simulink model "VelocidadeComoEntradaNoBlocoMotor"  (R2024b)
settings: Solver=VariableStepAuto  StartTime=0.0  StopTime=10  RelTol=1e-3
undefined symbols (not defined in the file): AirTemperature, C1, C2, C3, EV, fractalcoef, MTR, VelRef
libraries: vehdynlibtire x4, autolibmappedmotor x2, vrlib x1, slpidlib x1, mspsensorlib x1, vehdynlibviscommon x1, vehdynlibscenariocommon x1, vehdynlibsuspension x1, vehdynlibsteering x1, vehdynlibdriver x1, autolibshared x1
(part 1 of 3)
settings Model: SimulationMode=accelerator  Creator=João Gabriel  LastModifiedBy=João Gabriel
settings SolverCC: ZeroCrossAlgorithm=Adaptive
settings DebuggingCC: IgnoredZcDiagnostic=none

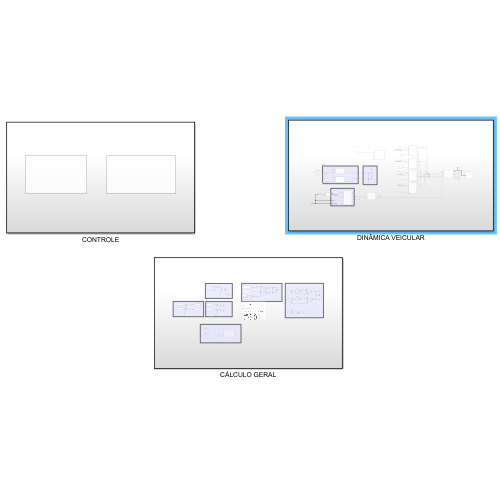
[thumbnail: Simulink's stored preview of the top-level diagram]
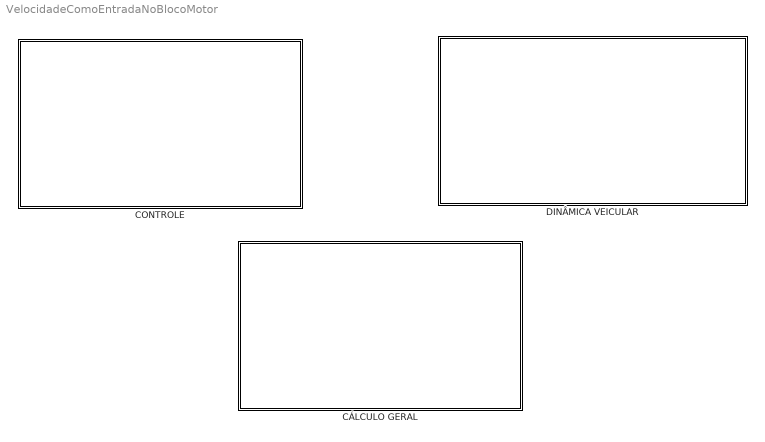
== system VelocidadeComoEntradaNoBlocoMotor ==
  CONTROLE : Subsystem
  CÁLCULO GERAL : Subsystem
  DINÂMICA VEICULAR : Subsystem

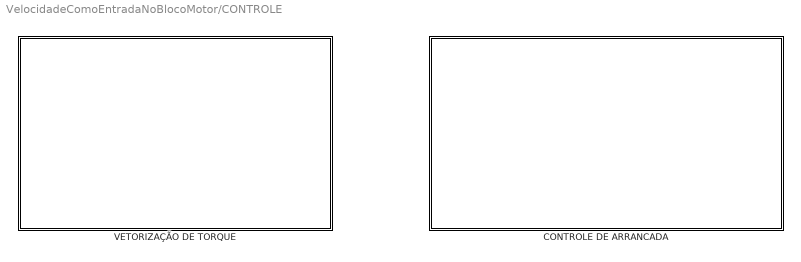
== system VelocidadeComoEntradaNoBlocoMotor/CONTROLE ==
  "CONTROLE DE ARRANCADA " : Subsystem
  "VETORIZAÇÃO DE TORQUE " : Subsystem

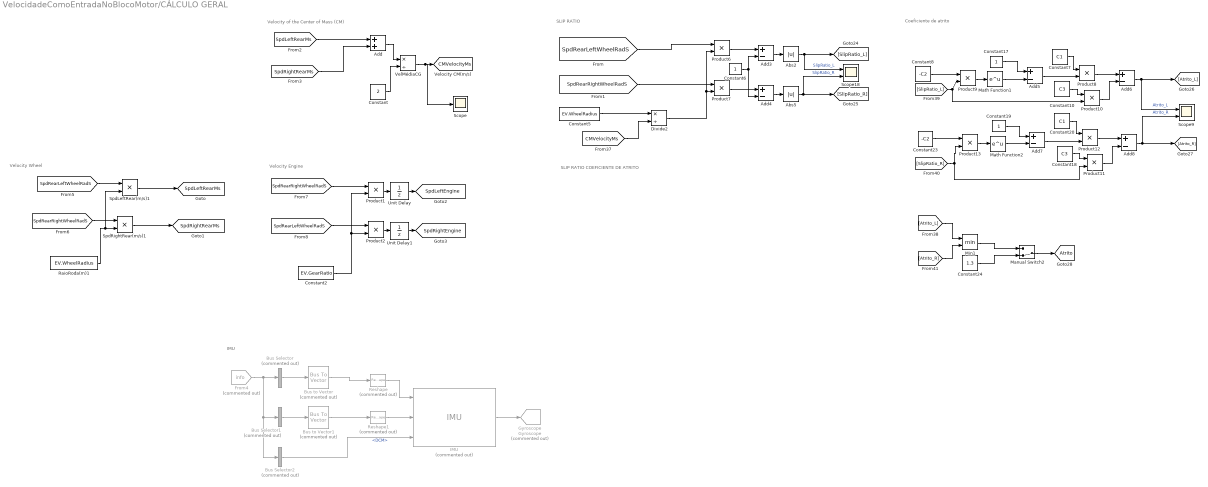
== system VelocidadeComoEntradaNoBlocoMotor/CÁLCULO GERAL ==
  note: Velocity Wheel
  note: Velocity Engine
  note: IMU
  note: Velocity of the Center of Mass (CM)
  note: SLIP RATIO
  note: Coeficiente de atrito
  note: SLIP RATIO
      |
      | COEFICIENTE DE ATRITO
  Abs2 : Abs  SaturateOnIntegerOverflow=off
  Abs5 : Abs  SaturateOnIntegerOverflow=off
  Add : Sum
  Add{3..8} (6 alike) : Sum  Inputs=+-
  Bus Selector : BusSelector  Commented=on  OutputSignals=BdyFrm.Cg.Acc.zddot,BdyFrm.Cg.Acc.yddot,BdyFrm.Cg.Acc.xddot  OutputAsBus=on
  Bus Selector1 : BusSelector  Commented=on  OutputSignals=BdyFrm.Cg.AngVel.p,BdyFrm.Cg.AngVel.q,BdyFrm.Cg.AngVel.r  OutputAsBus=on
  Bus Selector2 : BusSelector  Commented=on  OutputSignals=BdyFrm.Cg.DCM
  Bus to Vector : BusToVector  Commented=on
  Bus to Vector1 : BusToVector  Commented=on
  Constant : Constant  Value=2
  Constant10 : Constant  Value=C3
  Constant17 : Constant
  Constant18 : Constant  Value=C3
  Constant19 : Constant
  Constant2 : Constant  Value=EV.GearRatio
  Constant20 : Constant  Value=C1
  Constant23 : Constant  Value=-C2
  Constant24 : Constant  Value=1.3  VectorParams1D=off
  Constant5 : Constant  Value=EV.WheelRadius  VectorParams1D=off
  Constant6 : Constant
  Constant7 : Constant  Value=C1
  Constant8 : Constant  Value=-C2
  Divide2 : Product  Inputs=*/
  From4 : From  Commented=on  GotoTag=info  TagVisibility=global
  "Gyroscope " : Goto  Commented=on  GotoTag=Gyroscope  TagVisibility=global
  IMU : mspsensorlib/IMU  Commented=on  DispRefFrame=NED  TemperaturePort=off  Temperature=25  MagneticFieldPort=off  MagneticFieldNED=[ 27.5550, -2.4169, -16.0849 ]  MagneticFieldENU=[ -2.4169, 27.5550, 16.0849 ]  SeedDouble=67  SimulateUsing=Interpreted execution  AccelParamsMeasurementRange=Inf  AccelParamsResolution=0  AccelParamsConstantBias=[ 0, 0, 0 ]  AccelParamsAxesMisalignment=[ 100, 0, 0; 0, 100, 0; 0, 0, 100 ]  AccelParamsNoiseDensity=[ 0, 0, 0 ]  AccelParamsBiasInstability=[ 0, 0, 0 ]  AccelParamsBiasInstabilityNumerator=fractalcoef().Numerator  AccelParamsBiasInstabilityDenominator=fractalcoef().Denominator  AccelParamsRandomWalk=[ 0, 0, 0 ]  AccelParamsNoiseType=double-sided  AccelParamsTemperatureBias=[ 0, 0, 0 ]  AccelParamsTemperatureScaleFactor=[ 0, 0, 0 ]  GyroParamsMeasurementRange=Inf  GyroParamsResolution=0  GyroParamsConstantBias=[ 0, 0, 0 ]  GyroParamsAxesMisalignment=[ 100, 0, 0; 0, 100, 0; 0, 0, 100 ]  GyroParamsAccelerationBias=[ 0, 0, 0 ]  GyroParamsNoiseDensity=[ 0, 0, 0 ]  GyroParamsBiasInstability=[ 0, 0, 0 ]  GyroParamsBiasInstabilityNumerator=fractalcoef().Numerator  GyroParamsBiasInstabilityDenominator=fractalcoef().Denominator  GyroParamsRandomWalk=[ 0, 0, 0 ]  GyroParamsNoiseType=double-sided  GyroParamsTemperatureBias=[ 0, 0, 0 ]  GyroParamsTemperatureScaleFactor=[ 0, 0, 0 ]  MagParamsMeasurementRange=Inf  MagParamsResolution=0  MagParamsConstantBias=[ 0, 0, 0 ]  MagParamsAxesMisalignment=[ 100, 0, 0; 0, 100, 0; 0, 0, 100 ]  MagParamsNoiseDensity=[ 0, 0, 0 ]  MagParamsBiasInstability=[ 0, 0, 0 ]  MagParamsBiasInstabilityNumerator=fractalcoef().Numerator  MagParamsBiasInstabilityDenominator=fractalcoef().Denominator  MagParamsRandomWalk=[ 0, 0, 0 ]  MagParamsNoiseType=double-sided  MagParamsTemperatureBias=[ 0, 0, 0 ]  MagParamsTemperatureScaleFactor=[ 0, 0, 0 ]
  Manual Switch2 : ManualSwitch  CurrentSetting=0
  Math Function1 : Math
  Math Function2 : Math
  Min1 : MinMax  Inputs=2
  Product{1..2,6..13} (10 alike) : Product
  RaioRoda(m)1 : Constant  Value=EV.WheelRadius  VectorParams1D=off
  Reshape : Reshape  Commented=on  OutputDimensionality=Customize  OutputDimensions=[1,3]
  Reshape1 : Reshape  Commented=on  OutputDimensionality=Customize  OutputDimensions=[1,3]
  Scope : Scope
  Scope18 : Scope  NumInputPorts=2
  Scope9 : Scope  NumInputPorts=2
  SpdLeftRear(m/s)1 : Product
  SpdRightRear(m/s)1 : Product
  Unit Delay : UnitDelay  SampleTime=-1  HasFrameUpgradeWarning=on
  Unit Delay1 : UnitDelay  SampleTime=-1  HasFrameUpgradeWarning=on
  VelMédiaCG : Product  Inputs=*/
  tag scope: Atrito=global, CMVelocityMs=global, SpdLeftEngine=global, SpdLeftRearMs=global, SpdRightEngine=global, SpdRightRearMs=global
  wires:
  Constant6/1 -> Add3/2, Add4/2
  Add6/1 -> Scope9/1, [Atrito_L]  "Atrito_L"
  Abs2/1 -> Scope18/1, [SlipRatio_L]  "SlipRatio_L"
  Constant7/1 -> Product8/1
  Constant19/1 -> Add7/1
  Constant24/1 -> Manual Switch2/2
  Constant23/1 -> Product13/1
  Add4/1 -> Abs5/1
  Add3/1 -> Abs2/1
  Product11/1 -> Add8/2
  Abs5/1 -> Scope18/2, [SlipRatio_R]  "SlipRatio_R"
  Product12/1 -> Add8/1
  Product10/1 -> Add6/2
  Product8/1 -> Add6/1
  Math Function2/1 -> Add7/2
  Add7/1 -> Product12/2
  [Atrito_L] -> Min1/1
  Constant10/1 -> Product10/1
  Math Function1/1 -> Add5/2
  Constant18/1 -> Product11/1
  [SlipRatio_L] -> Product10/2, Product9/2
  Add8/1 -> Scope9/2, [Atrito_R]  "Atrito_R"
  Product9/1 -> Math Function1/1
  [CMVelocityMs] -> Divide2/2
  Min1/1 -> Manual Switch2/1
  Constant8/1 -> Product9/1
  Constant17/1 -> Add5/1
  [Atrito_R] -> Min1/2
  Constant5/1 -> Divide2/1
  Divide2/1 -> Product6/2, Product7/2
  Product13/1 -> Math Function2/1
  Constant20/1 -> Product12/1
  Product7/1 -> Add4/1
  Add5/1 -> Product8/2
  [SlipRatio_R] -> Product13/2, Product11/2
  Product6/1 -> Add3/1
  Manual Switch2/1 -> [Atrito]
  [SpdRearRightWheelRadS] -> Product7/1
  [SpdRearLeftWheelRadS] -> Product6/1
  Add/1 -> VelMédiaCG/1
  Constant/1 -> VelMédiaCG/2
  VelMédiaCG/1 -> Scope/1, [CMVelocityMs]
  From4/1 -> Bus Selector2/1, Bus Selector1/1, Bus Selector/1
  Bus Selector2/1 -> IMU/3  "<DCM>"
  IMU/2 -> "Gyroscope "/1
  Bus Selector/1 -> Bus to Vector/1
  Bus to Vector/1 -> Reshape/1
  Reshape/1 -> IMU/1
  Bus Selector1/1 -> Bus to Vector1/1
  Bus to Vector1/1 -> Reshape1/1
  Reshape1/1 -> IMU/2
  RaioRoda(m)1/1 -> SpdLeftRear(m/s)1/2, SpdRightRear(m/s)1/2
  SpdLeftRear(m/s)1/1 -> [SpdLeftRearMs]
  SpdRightRear(m/s)1/1 -> [SpdRightRearMs]
  [SpdRightRearMs] -> Add/2
  [SpdLeftRearMs] -> Add/1
  Constant2/1 -> Product2/2, Product1/2
  [SpdRearRightWheelRadS] -> Product1/1
  [SpdRearLeftWheelRadS] -> Product2/1
  [SpdRearLeftWheelRadS] -> SpdLeftRear(m/s)1/1
  [SpdRearRightWheelRadS] -> SpdRightRear(m/s)1/1
  Product1/1 -> Unit Delay/1
  Unit Delay/1 -> [SpdLeftEngine]
  Product2/1 -> Unit Delay1/1
  Unit Delay1/1 -> [SpdRightEngine]
